simulink model "untitled"  (R2019a)
settings: Solver=VariableStepAuto  StartTime=0.0  StopTime=30  RelTol=1e-3
settings Model: Creator=91516  LastModifiedBy=91516

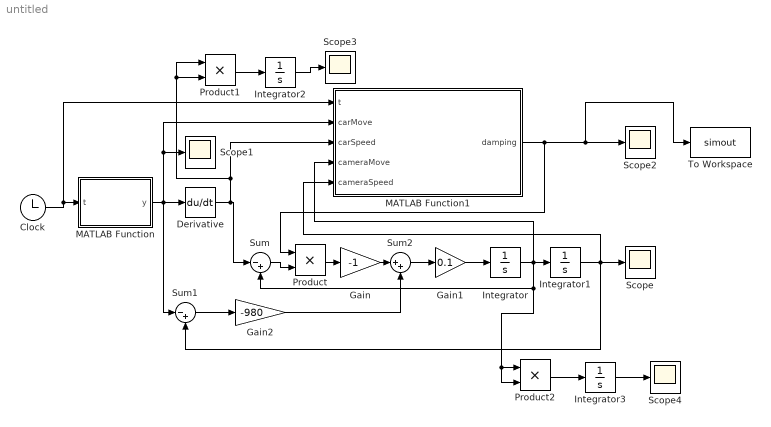
== system untitled ==
  Clock : Clock
      settings: Decimation=1000
  Derivative : Derivative  CoefficientInTFapproximation=0
  Gain : Gain  Gain=-1
  Gain1 : Gain  Gain=0.1
  Gain2 : Gain  Gain=-980
  Integrator{,1..3} (4 alike) : Integrator
  MATLAB Function : MATLAB Function  TreatAsAtomicUnit=on
  MATLAB Function1 : MATLAB Function  TreatAsAtomicUnit=on
  Product : Product
  Product1 : Product
  Product2 : Product
  Scope{,1..4} (5 alike) : Scope
  Sum : Sum  Inputs=|-+
  Sum1 : Sum  Inputs=|-+
  Sum2 : Sum  Inputs=|++
  To Workspace : ToWorkspace  VariableName=simout  SaveFormat=Timeseries  SampleTime=-1
  wires:
  Clock/1 -> MATLAB Function1/1(t), MATLAB Function/1(t)
  MATLAB Function/1(y) -> MATLAB Function1/2(carMove), Scope1/1, Sum1/1, Derivative/1
  Derivative/1 -> Product1/1, Product1/2, MATLAB Function1/3(carSpeed), Sum/1
  Sum/1 -> Product/2
  Integrator1/1 -> MATLAB Function1/5(cameraSpeed), Scope/1, Sum1/2
  Sum1/1 -> Gain2/1
  Gain2/1 -> Sum2/2
  Sum2/1 -> Gain1/1
  Gain1/1 -> Integrator/1
  Integrator/1 -> Product2/2, Product2/1, Sum/2, MATLAB Function1/4(cameraMove), Integrator1/1
  MATLAB Function1/1(damping) -> Product/1, To Workspace/1, Scope2/1
  Product/1 -> Gain/1
  Gain/1 -> Sum2/1
  Product1/1 -> Integrator2/1
  Integrator2/1 -> Scope3/1
  Product2/1 -> Integrator3/1
  Integrator3/1 -> Scope4/1

== matlab function untitled/MATLAB Function1 ==
  data: t input; damping output size=1; carMove input; carSpeed input; cameraMove input; cameraSpeed input
function damping = calculateDamping(t,carMove,carSpeed,cameraMove,cameraSpeed)
    speed=5;
    idealMove=5*sin(t*speed/20);
    k=980;
    idealDampingCofficient=10;
    idealForce=idealDampingCofficient*(idealMove-cameraMove)*10;
    idealDampingForce=idealForce+k*(cameraMove-carMove);
    if cameraSpeed ~= carSpeed
        idealDamping = -idealDampingForce/(cameraSpeed-carSpeed);
    else
        idealDamping=-600;
    end
     if idealDamping>=-600
         idealDamping=-600;
     end
    if idealDamping<=-2400
        idealDamping=-2400;
    end
    damping=-idealDamping;
     damping=1000;
end

== matlab function untitled/MATLAB Function ==
  data: t input; y output
function y  = getRandomRoad(t)
%UNTITLED 此处显示有关此函数的摘要
%   此处显示详细说明
speed=3;
 y=5*sin(t*speed/20)+0.5*sin(t*speed/4)+0.3*sin(t*speed*6)+0.02*sin(t*speed*30)+0.3*sin(t*speed*60);
%     if rem(t,4)<2
%         y=5*sin(t*speed/20)+0.5*sin(t*speed/4)+0.3*sin(t*speed*6)+0.02*sin(t*speed*30)+0.3*sin(t*speed*60);
%     else
%         y=5*sin(t*speed/20)+0.5*sin(t*speed/4);
%     end
%y=sin(t*5*6.28);
end
